simulink model "real2bytes"  (R2016b)
settings: Solver=VariableStepAuto  StartTime=0.0  StopTime=10.0  RelTol=1e-3
settings Model: Creator=mhussa27  LastModifiedBy=mhussa27

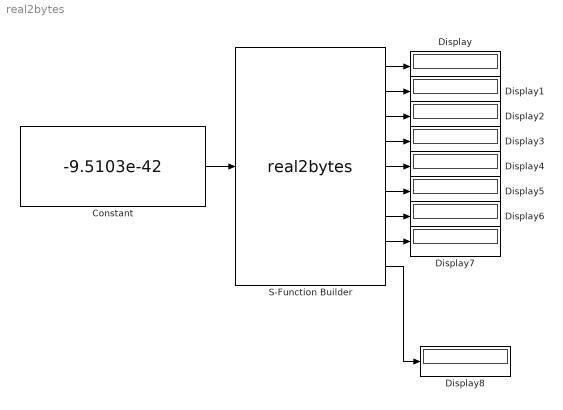
== system real2bytes ==
  Constant : Constant  Value=-9.5103e-42  OutDataTypeStr=double
  Display{,1..8} (9 alike) : Display
  S-Function Builder : S-Function  InitFcn=try, set_param(gcb,'FunctionName','real2bytes'), end  FunctionName=real2bytes  SFunctionModules=real2bytes_wrapper  SFunctionDeploymentMode=off  EnableBusSupport=off  mask(S-Function Builder){}
      mask help: Simulink:masks:SFunctionBuilder_MD
      mask init:
      | val = [[.9  0.75 0.75 1 1 .9 .9 1]',[1 1 0.75 0.75 .9 .9 1 .9]'];try , sys = get_param(gcb,'SfunBuilderFcnName');if isempty(sys), sys = get_param(gcb,'FunctionName'); end,catch, sys = get_param(gcb,'FunctionName'); end
      settings: CopyFcn=set_param(gcbh,'LinkStatus','none')  PreSaveFcn=try, set_param(gcb,'FunctionName','real2bytes'), end  OpenFcn=sfunctionwizard(gcbh)
      mask Display: plot(val(:,1),val(:,2)),disp(sys), port_label('input',1,'u0'), port_label('output',1,'y0'), port_label('output',2,'y1'), port_label('output',3,'y2'), port_label('output',4,'y3'), port_label('output',5,'y4'), port_label('output',6,'y5'), port_label('output',7,'y6'), port_label('output',8,'y7'), port_label('output',9,'size')
  wires:
  Constant/1 -> S-Function Builder/1
  S-Function Builder/1 -> Display/1
  S-Function Builder/2 -> Display1/1
  S-Function Builder/3 -> Display2/1
  S-Function Builder/4 -> Display3/1
  S-Function Builder/5 -> Display4/1
  S-Function Builder/6 -> Display5/1
  S-Function Builder/7 -> Display6/1
  S-Function Builder/8 -> Display7/1
  S-Function Builder/9 -> Display8/1
